simulink model "Car_sliding_modified"  (R2020a)
settings: Solver=FixedStepAuto  StartTime=0.0  StopTime=20  FixedStep=1e-4  RelTol=1e-3  EnableMultiTasking=on
settings Model: Creator=ayyrao  LastModifiedBy=nikhil
settings SolverCC: MaxConsecutiveMinStep=4
settings DataIOCC: LimitDataPoints=on  SaveFormat=Array  ReturnWorkspaceOutputs=off
settings OptimizationCC: LifeSpan=inf
settings DebuggingCC: SFUnexpectedBacktrackingDiag=warning  SFNoUnconditionalDefaultTransitionDiag=warning  SFExecutionAtInitializationDiag=none  ArithmeticOperatorsInVariantConditions=warning
settings HardwareCC: ProdBitPerPointer=32  ProdBitPerSizeT=32  ProdBitPerPtrDiffT=32  ProdLargestAtomicFloat=None  ProdIntDivRoundTo=Undefined  ProdEndianess=Unspecified  ProdWordSize=32  ProdHWDeviceType=32-bit Generic
settings ModelReferenceCC: PropagateSignalLabelsOutOfModel=off
settings SFSimCC: SimUseLocalCustomCode=off  CustomCodeUndefinedFunction=UseInterfaceOnly
settings RTWCC: RTWUseLocalCustomCode=off
settings CodeAppCC: StateflowObjectComments=on
settings GRTTargetCC: TargetLangStandard=C89/C90 (ANSI)
settings ConfigComp: CovMetricSettings=dw  CovHtmlReporting=on  CovSaveCumulativeToWorkspaceVar=on  CovSaveSingleToWorkspaceVar=on  CovExternalEMLEnable=off

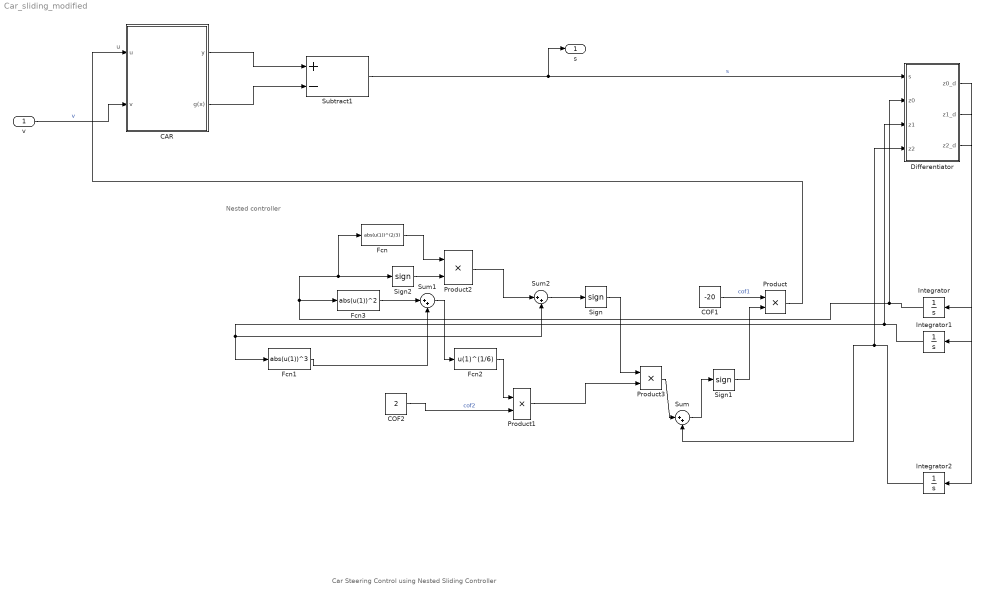
== system Car_sliding_modified ==
  note: Nested controller
  note: u
  note: Car Steering Control using Nested Sliding Controller
  v : Inport
  CAR : Subsystem
      mask Display: image('ferrari-488-spider.jpg');
  COF1 : Constant  Value=-20
  COF2 : Constant  Value=2
  Differentiator : MATLAB Function  TreatAsAtomicUnit=on
  Fcn : Fcn  Expr=abs(u(1))^(2/3)
  Fcn1 : Fcn  Expr=abs(u(1))^3
  Fcn2 : Fcn  Expr=u(1)^(1/6)
  Fcn3 : Fcn  Expr=abs(u(1))^2
  Integrator : Integrator
  Integrator1 : Integrator
  Integrator2 : Integrator
  Product{,1..3} (4 alike) : Product
  Sign : Signum
  Sign1 : Signum
  Sign2 : Signum
  Subtract1 : Sum  Inputs=+-
  Sum : Sum  Inputs=|++
  Sum1 : Sum  Inputs=|++
  Sum2 : Sum  Inputs=|++
  s : Outport
  wires:
  CAR/1(y) -> Subtract1/1
  CAR/2(g(x)) -> Subtract1/2
  Subtract1/1 -> Differentiator/1(s), s/1  "s"
  Differentiator/1(z0_d) -> Integrator/1
  Differentiator/2(z1_d) -> Integrator1/1
  Differentiator/3(z2_d) -> Integrator2/1
  Product/1 -> CAR/1(u)
  ? -> ?
  v/1 -> CAR/2(v)  "v"
  Fcn2/1 -> Product1/1
  Sign1/1 -> Product/2
  Product3/1 -> Sum/1
  Sum2/1 -> Sign/1
  Product2/1 -> Sum2/1
  Fcn/1 -> Product2/1
  Sign2/1 -> Product2/2
  Product1/1 -> Product3/2
  Sum/1 -> Sign1/1
  COF2/1 -> Product1/2  "cof2"
  Sum1/1 -> Fcn2/1
  Fcn1/1 -> Sum1/2
  Fcn3/1 -> Sum1/1
  Integrator1/1 -> Fcn1/1, Sum2/2, Differentiator/3(z1)
  Integrator/1 -> Fcn3/1, Fcn/1, Sign2/1, Differentiator/2(z0)
  Integrator2/1 -> Sum/2, Differentiator/4(z2)
  Sign/1 -> Product3/1
  COF1/1 -> Product/1  "cof1"

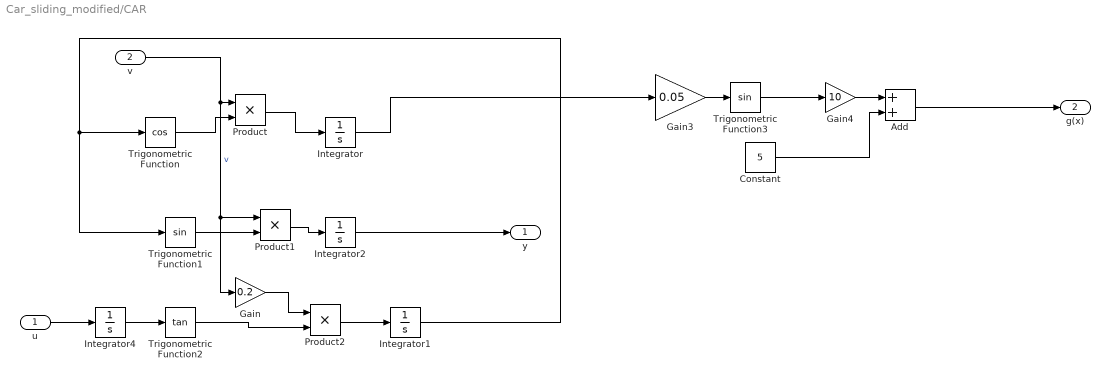
== system Car_sliding_modified/CAR ==
  u : Inport
  v : Inport  Port=2
  Add : Sum
  Constant : Constant  Value=5
  Gain : Gain  Gain=0.2
  Gain3 : Gain  Gain=0.05
  Gain4 : Gain  Gain=10
  Integrator{,1..2,4} (4 alike) : Integrator
  Product : Product
  Product1 : Product
  Product2 : Product
  Trigonometric Function : Trigonometry  Operator=cos
  Trigonometric Function1 : Trigonometry
  Trigonometric Function2 : Trigonometry  Operator=tan
  Trigonometric Function3 : Trigonometry
  y : Outport  VectorParamsAs1DForOutWhenUnconnected=off
  g(x) : Outport  Port=2  VectorParamsAs1DForOutWhenUnconnected=off
  wires:
  Product/1 -> Integrator/1
  Trigonometric Function/1 -> Product/2
  Trigonometric Function1/1 -> Product1/2
  Product1/1 -> Integrator2/1
  Trigonometric Function2/1 -> Product2/2
  Product2/1 -> Integrator1/1
  Integrator1/1 -> Trigonometric Function1/1, Trigonometric Function/1
  Gain3/1 -> Trigonometric Function3/1
  Trigonometric Function3/1 -> Gain4/1
  Gain4/1 -> Add/1
  Constant/1 -> Add/2
  Integrator/1 -> Gain3/1
  Integrator2/1 -> y/1
  Add/1 -> g(x)/1
  v/1 -> Gain/1, Product1/1, Product/1  "v"
  Gain/1 -> Product2/1
  Integrator4/1 -> Trigonometric Function2/1
  u/1 -> Integrator4/1

== matlab function Car_sliding_modified/Differentiator ==
  data: s input; z0 input; z1 input; z2 input; z0_d output; z1_d output; z2_d output
function [z0_d,z1_d,z2_d]= fcn(s,z0,z1,z2)
%%% JKD Power and Energy solutions
%% Differentiator
v0 = -14.7361*(abs(z0-s))^(2/3)*sign(z0-s)+z1;
v1 = -30*(abs(z1-v0))^(1/2)*sign(z1-v0)+z2;
z0_d = v0;
z1_d  = v1;
z2_d  = -400*sign(z2-v1);
end
